simulink model "RealimentacaoIntegralComObservadorPadrao"  (R2019a)
settings: Solver=VariableStepAuto  StartTime=0.0  StopTime=10  RelTol=1e-3
undefined symbols (not defined in the file): A, B, C, K, Ke, L
settings Model: Creator=Cliente  LastModifiedBy=Cliente

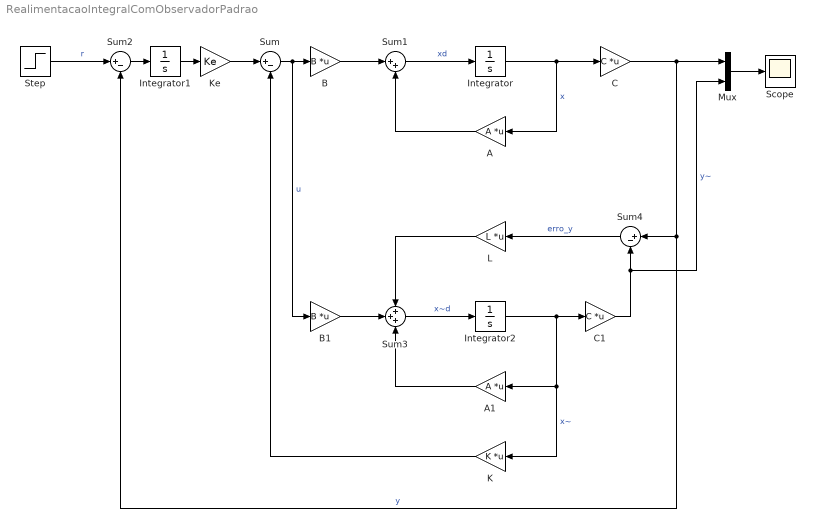
== system RealimentacaoIntegralComObservadorPadrao ==
  A : Gain  Gain=A  Multiplication=Matrix(K*u) (u vector)
  A1 : Gain  Gain=A  Multiplication=Matrix(K*u) (u vector)
  B : Gain  Gain=B  Multiplication=Matrix(K*u)
  B1 : Gain  Gain=B  Multiplication=Matrix(K*u)
  C : Gain  Gain=C  Multiplication=Matrix(K*u) (u vector)
  C1 : Gain  Gain=C  Multiplication=Matrix(K*u) (u vector)
  Integrator : Integrator
  Integrator1 : Integrator
  Integrator2 : Integrator
  K : Gain  Gain=K  Multiplication=Matrix(K*u) (u vector)
  Ke : Gain  Gain=Ke
  L : Gain  Gain=L  Multiplication=Matrix(K*u)
  Mux : Mux  Inputs=2
  Scope : Scope
  Step : Step  Time=0  SampleTime=0
  Sum : Sum  Inputs=|+-
  Sum1 : Sum  Inputs=|++
  Sum2 : Sum  Inputs=|+-
  Sum3 : Sum  Inputs=+++
  Sum4 : Sum  Inputs=|+-
  wires:
  Integrator/1 -> A/1, C/1  "x"
  C/1 -> Mux/1, Sum4/1, Sum2/2  "y"
  Sum1/1 -> Integrator/1  "xd"
  B/1 -> Sum1/1
  Sum/1 -> B1/1, B/1  "u"
  Step/1 -> Sum2/1  "r"
  A/1 -> Sum1/2
  K/1 -> Sum/2
  Sum2/1 -> Integrator1/1
  Integrator1/1 -> Ke/1
  Ke/1 -> Sum/1
  Integrator2/1 -> K/1, A1/1, C1/1  "x~"
  Sum3/1 -> Integrator2/1  "x~d"
  C1/1 -> Mux/2, Sum4/2  "y~"
  Mux/1 -> Scope/1
  Sum4/1 -> L/1  "erro_y"
  A1/1 -> Sum3/3
  B1/1 -> Sum3/2
  L/1 -> Sum3/1
